simulink model "reg02"  (Simulink 4.00)
settings: Solver=ode45  StartTime=0.0  StopTime=40  MaxStep=0.05  MinStep=0.01  RelTol=1e-3  AbsTol=1e-3
values from neighbouring files (symbols this model uses):
  Kp = X(1)    [eval_reg02.m]    (also in eval_reg06.m)
  Td = X(3)    [eval_reg02.m]    (also in eval_reg06.m)
  Ti = X(2)    [eval_reg02.m]    (also in eval_reg06.m)
settings Model: LastModifiedBy=LPEE_Plamen  SaveTime=off  SaveOutput=off  BlockReductionOpt=off

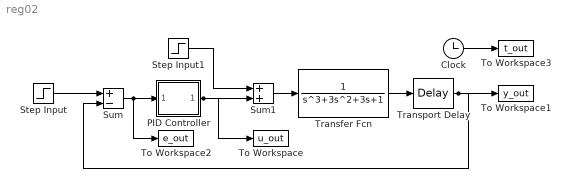
== system reg02 ==
  Clock : Clock
      settings: DisplayTime=off  Decimation=10
  PID Controller : Subsystem
      settings: RTWFcnNameOpts=Auto  RTWFileNameOpts=Auto
  Step Input : Step  Time=0  Before=0  After=1  SampleTime=0
  Step Input1 : Step  Time=60  Before=0  After=0  SampleTime=0
  Sum : Sum  Inputs=+-  SaturateOnIntegerOverflow=on
  Sum1 : Sum  Inputs=++  SaturateOnIntegerOverflow=on
  To Workspace : ToWorkspace  VariableName=u_out  SampleTime=-1  SaveFormat=Array
  To Workspace1 : ToWorkspace  VariableName=y_out  SampleTime=-1  SaveFormat=Array
  To Workspace2 : ToWorkspace  VariableName=e_out  SampleTime=-1  SaveFormat=Array
  To Workspace3 : ToWorkspace  VariableName=t_out  SampleTime=-1  SaveFormat=Array
  Transfer Fcn : TransferFcn  Numerator=[1]  Denominator=[1 3 3 1]  Realization=auto  AbsoluteTolerance=auto
  Transport Delay : TransportDelay  DelayTime=5  InitialInput=0  BufferSize=10240  PadeOrder=0
  wires:
  Transfer Fcn/1 -> Transport Delay/1
  Sum/1 -> PID Controller/1(In_1), To Workspace2/1
  Step Input/1 -> Sum/1
  Sum1/1 -> Transfer Fcn/1
  Step Input1/1 -> Sum1/1
  PID Controller/1(Out_1) -> Sum1/2, To Workspace/1
  Transport Delay/1 -> To Workspace1/1, Sum/2
  Clock/1 -> To Workspace3/1

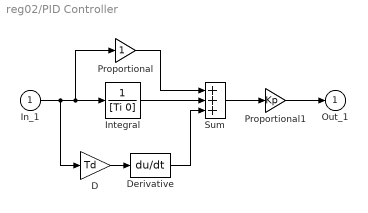
== system reg02/PID Controller ==
  In_1 : Inport  Port=1
  D : Gain  Gain=Td  Multiplication=Element-wise(K.*u)  SaturateOnIntegerOverflow=on
  Derivative : Derivative
  Integral : TransferFcn  Numerator=[1]  Denominator=[Ti 0]  Realization=auto  AbsoluteTolerance=auto
  Proportional : Gain  Gain=1  Multiplication=Element-wise(K.*u)  SaturateOnIntegerOverflow=on
  Proportional1 : Gain  Gain=Kp  Multiplication=Element-wise(K.*u)  SaturateOnIntegerOverflow=on
  Sum : Sum  Inputs=+++  SaturateOnIntegerOverflow=on
  Out_1 : Outport  Port=1
  wires:
  Proportional/1 -> Sum/1
  Integral/1 -> Sum/2
  Derivative/1 -> Sum/3
  In_1/1 -> Integral/1, Proportional/1, D/1
  D/1 -> Derivative/1
  Sum/1 -> Proportional1/1
  Proportional1/1 -> Out_1/1
